simulink model "untitled"  (R2021a)
settings: Solver=VariableStepAuto  StartTime=0.0  StopTime=10.0  RelTol=1e-3
undefined symbols (not defined in the file): period
libraries: dsparch4 x4
settings Model: Creator=sunshi1  LastModifiedBy=sunshi1

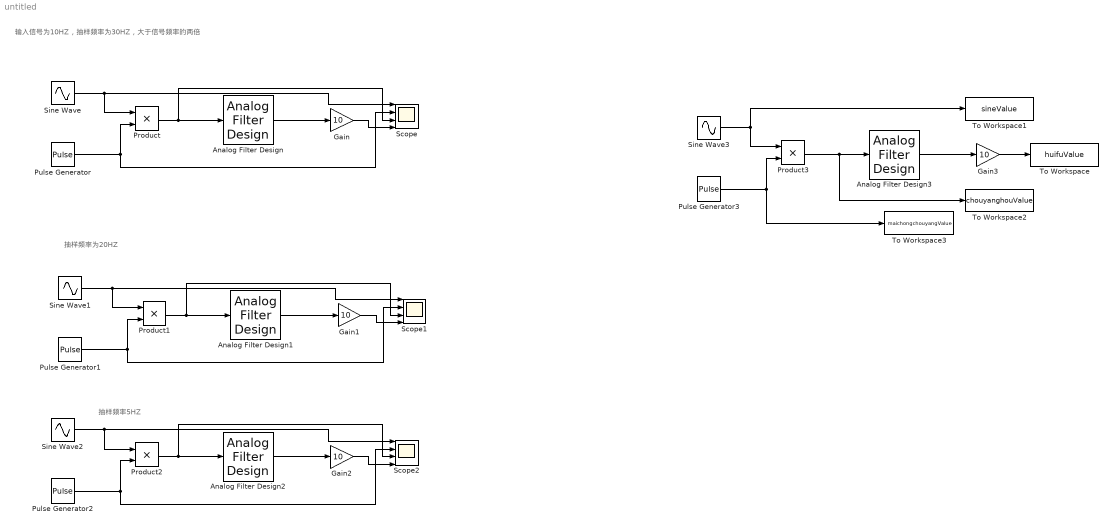
== system untitled ==
  note: 抽样频率5HZ
  note: 抽样频率为20HZ
  note: 输入信号为10HZ，抽样频率为30HZ，大于信号频率的两倍
  Analog Filter Design{,1..3} (4 alike) : dsparch4/Analog Filter Design  method=Butterworth  filttype=Lowpass  N=8  Wlo=24*pi  Whi=80  Rp=2  Rs=40
  Gain{,1..3} (4 alike) : Gain  Gain=10
  Product{,1..3} (4 alike) : Product
  Pulse Generator : DiscretePulseGenerator  PulseType=Time based  Period=1/30  PulseWidth=10
  Pulse Generator1 : DiscretePulseGenerator  PulseType=Time based  Period=0.05  PulseWidth=10
  Pulse Generator2 : DiscretePulseGenerator  PulseType=Time based  Period=0.2  PulseWidth=10
  Pulse Generator3 : DiscretePulseGenerator  PulseType=Time based  Period=1/period  PulseWidth=10
  Scope : Scope  NumInputPorts=4
  Scope1 : Scope  NumInputPorts=4
  Scope2 : Scope  NumInputPorts=4
  Sine Wave{,1..3} (4 alike) : Sin  Frequency=20*pi  SampleTime=0
  To Workspace : ToWorkspace  VariableName=huifuValue  SaveFormat=Timeseries  SampleTime=-1
  To Workspace1 : ToWorkspace  VariableName=sineValue  SaveFormat=Timeseries  SampleTime=-1
  To Workspace2 : ToWorkspace  VariableName=chouyanghouValue  SaveFormat=Timeseries  SampleTime=-1
  To Workspace3 : ToWorkspace  VariableName=maichongchouyangValue  SaveFormat=Timeseries  SampleTime=-1
  wires:
  Sine Wave/1 -> Scope/1, Product/1
  Pulse Generator/1 -> Scope/2, Product/2
  Product/1 -> Scope/3, Analog Filter Design/1
  Analog Filter Design/1 -> Gain/1
  Gain/1 -> Scope/4
  Gain1/1 -> Scope1/4
  Product1/1 -> Scope1/3, Analog Filter Design1/1
  Pulse Generator1/1 -> Scope1/2, Product1/2
  Sine Wave1/1 -> Scope1/1, Product1/1
  Analog Filter Design1/1 -> Gain1/1
  Gain2/1 -> Scope2/4
  Product2/1 -> Scope2/3, Analog Filter Design2/1
  Pulse Generator2/1 -> Scope2/2, Product2/2
  Sine Wave2/1 -> Scope2/1, Product2/1
  Analog Filter Design2/1 -> Gain2/1
  Product3/1 -> To Workspace2/1, Analog Filter Design3/1
  Pulse Generator3/1 -> To Workspace3/1, Product3/2
  Sine Wave3/1 -> To Workspace1/1, Product3/1
  Analog Filter Design3/1 -> Gain3/1
  Gain3/1 -> To Workspace/1
